simulink model "uwb_re_blackbox"  (Simulink 8.0)
settings: Solver=ode45  StartTime=0.0  StopTime=330  RelTol=1e-3
InitFcn:
  | set_channel;
  | Int_Data_input;
StopFcn:
  | abc=1;
undefined symbols (not defined in the file or in its folder): rsgenpoly
libraries: commutil2 x88, simulink x53, dspmtrx3 x33, dspindex x16, xbsIndex_r4 x12, commcnvcod2 x8, commblkcod2 x8, dspsigops x2, commsink2 x2, commchan3 x1
(part 3 of 5)

== system uwb_re_blackbox/Subsystem2/Transmit2/Spreading/Hop3 ==
  data : Inport
  s : Inport  Port=2
  Gain2 : Gain  Gain=-1  OutDataTypeStr=int8
  Gain4 : Gain  Gain=-1  OutDataTypeStr=int8
  Kron : Subsystem
      mask Display:
      | disp('KRON');
      | 
      | port_label('input',1,'P');
      | port_label('input',2,'-P');
      | port_label('input',3,'sel');
      | port_label('output',1,'burst');
  Kron1 : Subsystem
      mask Display:
      | disp('KRON');
      | 
      | port_label('input',1,'S');
      | port_label('input',2,'-S');
      | port_label('input',3,'sel');
      | port_label('output',1,'signS');
  Subsystem2 : Subsystem
      mask Display: disp('1/2 Frame data pulse')
  Subsystem3 : Subsystem
      mask Display:
      | port_label('input',1,'data_conv');
      | port_label('output',2,'sign');
      | port_label('output',1,'position');
  Subsystem5 : Subsystem
      mask Display:
      | disp('sel position');
      | 
      | port_label('input',1,'position');
      | port_label('input',2,'matrix');
      | port_label('output',1,'mat_po');
  p : Constant  Value=[-0.0022 -0.0103 -0.0386 -0.1133 -0.2542 -0.4160 -0.4388 -0.1363 0.4543 0.9559 0.9559 0.4543 -0.1363 -0.4388 -0.4160 -0.2542 -0.1133 -0.0386 -0.0103 -0.0022]*2^6  VectorParams1D=off  OutDataTypeStr=int8
      mask Display: disp('xung P')
  Hop1 : Outport
  wires:
  data/1 -> Subsystem3/1(In1)
  Subsystem5/1(Out1) -> Hop1/1
  Subsystem3/1(position) -> Subsystem5/1(In1)
  Subsystem2/1(Out1) -> Subsystem5/2(matrix)
  Subsystem3/2(sign) -> Kron1/3(sel)
  s/1 -> Gain2/1, Kron1/1(p)
  Kron/1(burst) -> Subsystem2/1(In1)
  p/1 -> Gain4/1, Kron/1(p)
  Kron1/1(burst) -> Kron/3(sel)
  Gain4/1 -> Kron/2(-p)
  Gain2/1 -> Kron1/2(-p)

== system uwb_re_blackbox/Subsystem2/Transmit2/Spreading/Hop4 ==
  data : Inport
  s : Inport  Port=2
  Gain2 : Gain  Gain=-1  OutDataTypeStr=int8
  Gain4 : Gain  Gain=-1  OutDataTypeStr=int8
  Kron : Subsystem
      mask Display:
      | disp('KRON');
      | 
      | port_label('input',1,'P');
      | port_label('input',2,'-P');
      | port_label('input',3,'sel');
      | port_label('output',1,'burst');
  Kron1 : Subsystem
      mask Display:
      | disp('KRON');
      | 
      | port_label('input',1,'S');
      | port_label('input',2,'-S');
      | port_label('input',3,'sel');
      | port_label('output',1,'signS');
  Subsystem2 : Subsystem
      mask Display: disp('1/2 Frame data pulse')
  Subsystem3 : Subsystem
      mask Display:
      | port_label('input',1,'data_conv');
      | port_label('output',2,'sign');
      | port_label('output',1,'position');
  Subsystem5 : Subsystem
      mask Display:
      | disp('sel position');
      | 
      | port_label('input',1,'position');
      | port_label('input',2,'matrix');
      | port_label('output',1,'mat_po');
  p : Constant  Value=[-0.0022 -0.0103 -0.0386 -0.1133 -0.2542 -0.4160 -0.4388 -0.1363 0.4543 0.9559 0.9559 0.4543 -0.1363 -0.4388 -0.4160 -0.2542 -0.1133 -0.0386 -0.0103 -0.0022]*2^6  VectorParams1D=off  OutDataTypeStr=int8
      mask Display: disp('xung P')
  Hop1 : Outport
  wires:
  Gain2/1 -> Kron1/2(-p)
  Gain4/1 -> Kron/2(-p)
  Kron1/1(burst) -> Kron/3(sel)
  p/1 -> Kron/1(p), Gain4/1
  Kron/1(burst) -> Subsystem2/1(In1)
  s/1 -> Kron1/1(p), Gain2/1
  Subsystem3/2(sign) -> Kron1/3(sel)
  Subsystem2/1(Out1) -> Subsystem5/2(matrix)
  Subsystem3/1(position) -> Subsystem5/1(In1)
  Subsystem5/1(Out1) -> Hop1/1
  data/1 -> Subsystem3/1(In1)

== system uwb_re_blackbox/Subsystem2/Transmit2/Spreading/Hop5 ==
  data : Inport
  s : Inport  Port=2
  Gain2 : Gain  Gain=-1  OutDataTypeStr=int8
  Gain4 : Gain  Gain=-1  OutDataTypeStr=int8
  Kron : Subsystem
      mask Display:
      | disp('KRON');
      | 
      | port_label('input',1,'P');
      | port_label('input',2,'-P');
      | port_label('input',3,'sel');
      | port_label('output',1,'burst');
  Kron1 : Subsystem
      mask Display:
      | disp('KRON');
      | 
      | port_label('input',1,'S');
      | port_label('input',2,'-S');
      | port_label('input',3,'sel');
      | port_label('output',1,'signS');
  Subsystem2 : Subsystem
      mask Display: disp('1/2 Frame data pulse')
  Subsystem3 : Subsystem
      mask Display:
      | port_label('input',1,'data_conv');
      | port_label('output',2,'sign');
      | port_label('output',1,'position');
  Subsystem5 : Subsystem
      mask Display:
      | disp('sel position');
      | 
      | port_label('input',1,'position');
      | port_label('input',2,'matrix');
      | port_label('output',1,'mat_po');
  p : Constant  Value=[-0.0022 -0.0103 -0.0386 -0.1133 -0.2542 -0.4160 -0.4388 -0.1363 0.4543 0.9559 0.9559 0.4543 -0.1363 -0.4388 -0.4160 -0.2542 -0.1133 -0.0386 -0.0103 -0.0022]*2^6  VectorParams1D=off  OutDataTypeStr=int8
      mask Display: disp('xung P')
  Hop1 : Outport
  wires:
  data/1 -> Subsystem3/1(In1)
  Subsystem5/1(Out1) -> Hop1/1
  Subsystem3/1(position) -> Subsystem5/1(In1)
  Subsystem2/1(Out1) -> Subsystem5/2(matrix)
  Subsystem3/2(sign) -> Kron1/3(sel)
  s/1 -> Gain2/1, Kron1/1(p)
  Kron/1(burst) -> Subsystem2/1(In1)
  p/1 -> Gain4/1, Kron/1(p)
  Kron1/1(burst) -> Kron/3(sel)
  Gain4/1 -> Kron/2(-p)
  Gain2/1 -> Kron1/2(-p)

== system uwb_re_blackbox/Subsystem2/Transmit2/Spreading/Hop6 ==
  data : Inport
  s : Inport  Port=2
  Gain2 : Gain  Gain=-1  OutDataTypeStr=int8
  Gain4 : Gain  Gain=-1  OutDataTypeStr=int8
  Kron : Subsystem
      mask Display:
      | disp('KRON');
      | 
      | port_label('input',1,'P');
      | port_label('input',2,'-P');
      | port_label('input',3,'sel');
      | port_label('output',1,'burst');
  Kron1 : Subsystem
      mask Display:
      | disp('KRON');
      | 
      | port_label('input',1,'S');
      | port_label('input',2,'-S');
      | port_label('input',3,'sel');
      | port_label('output',1,'signS');
  Subsystem2 : Subsystem
      mask Display: disp('1/2 Frame data pulse')
  Subsystem3 : Subsystem
      mask Display:
      | port_label('input',1,'data_conv');
      | port_label('output',2,'sign');
      | port_label('output',1,'position');
  Subsystem5 : Subsystem
      mask Display:
      | disp('sel position');
      | 
      | port_label('input',1,'position');
      | port_label('input',2,'matrix');
      | port_label('output',1,'mat_po');
  p : Constant  Value=[-0.0022 -0.0103 -0.0386 -0.1133 -0.2542 -0.4160 -0.4388 -0.1363 0.4543 0.9559 0.9559 0.4543 -0.1363 -0.4388 -0.4160 -0.2542 -0.1133 -0.0386 -0.0103 -0.0022]*2^6  VectorParams1D=off  OutDataTypeStr=int8
      mask Display: disp('xung P')
  Hop1 : Outport
  wires:
  Gain2/1 -> Kron1/2(-p)
  Gain4/1 -> Kron/2(-p)
  Kron1/1(burst) -> Kron/3(sel)
  p/1 -> Kron/1(p), Gain4/1
  Kron/1(burst) -> Subsystem2/1(In1)
  s/1 -> Kron1/1(p), Gain2/1
  Subsystem3/2(sign) -> Kron1/3(sel)
  Subsystem2/1(Out1) -> Subsystem5/2(matrix)
  Subsystem3/1(position) -> Subsystem5/1(In1)
  Subsystem5/1(Out1) -> Hop1/1
  data/1 -> Subsystem3/1(In1)

== system uwb_re_blackbox/Subsystem2/Transmit2/Spreading/Hop7 ==
  data : Inport
  s : Inport  Port=2
  Gain2 : Gain  Gain=-1  OutDataTypeStr=int8
  Gain4 : Gain  Gain=-1  OutDataTypeStr=int8
  Kron : Subsystem
      mask Display:
      | disp('KRON');
      | 
      | port_label('input',1,'P');
      | port_label('input',2,'-P');
      | port_label('input',3,'sel');
      | port_label('output',1,'burst');
  Kron1 : Subsystem
      mask Display:
      | disp('KRON');
      | 
      | port_label('input',1,'S');
      | port_label('input',2,'-S');
      | port_label('input',3,'sel');
      | port_label('output',1,'signS');
  Subsystem2 : Subsystem
      mask Display: disp('1/2 Frame data pulse')
  Subsystem3 : Subsystem
      mask Display:
      | port_label('input',1,'data_conv');
      | port_label('output',2,'sign');
      | port_label('output',1,'position');
  Subsystem5 : Subsystem
      mask Display:
      | disp('sel position');
      | 
      | port_label('input',1,'position');
      | port_label('input',2,'matrix');
      | port_label('output',1,'mat_po');
  p : Constant  Value=[-0.0022 -0.0103 -0.0386 -0.1133 -0.2542 -0.4160 -0.4388 -0.1363 0.4543 0.9559 0.9559 0.4543 -0.1363 -0.4388 -0.4160 -0.2542 -0.1133 -0.0386 -0.0103 -0.0022]*2^6  VectorParams1D=off  OutDataTypeStr=int8
      mask Display: disp('xung P')
  Hop1 : Outport
  wires:
  data/1 -> Subsystem3/1(In1)
  Subsystem5/1(Out1) -> Hop1/1
  Subsystem3/1(position) -> Subsystem5/1(In1)
  Subsystem2/1(Out1) -> Subsystem5/2(matrix)
  Subsystem3/2(sign) -> Kron1/3(sel)
  s/1 -> Gain2/1, Kron1/1(p)
  Kron/1(burst) -> Subsystem2/1(In1)
  p/1 -> Gain4/1, Kron/1(p)
  Kron1/1(burst) -> Kron/3(sel)
  Gain4/1 -> Kron/2(-p)
  Gain2/1 -> Kron1/2(-p)

== system uwb_re_blackbox/Subsystem2/Transmit2/Spreading/Hop8 ==
  data : Inport
  s : Inport  Port=2
  Gain2 : Gain  Gain=-1  OutDataTypeStr=int8
  Gain4 : Gain  Gain=-1  OutDataTypeStr=int8
  Kron : Subsystem
      mask Display:
      | disp('KRON');
      | 
      | port_label('input',1,'P');
      | port_label('input',2,'-P');
      | port_label('input',3,'sel');
      | port_label('output',1,'burst');
  Kron1 : Subsystem
      mask Display:
      | disp('KRON');
      | 
      | port_label('input',1,'S');
      | port_label('input',2,'-S');
      | port_label('input',3,'sel');
      | port_label('output',1,'signS');
  Subsystem2 : Subsystem
      mask Display: disp('1/2 Frame data pulse')
  Subsystem3 : Subsystem
      mask Display:
      | port_label('input',1,'data_conv');
      | port_label('output',2,'sign');
      | port_label('output',1,'position');
  Subsystem5 : Subsystem
      mask Display:
      | disp('sel position');
      | 
      | port_label('input',1,'position');
      | port_label('input',2,'matrix');
      | port_label('output',1,'mat_po');
  p : Constant  Value=[-0.0022 -0.0103 -0.0386 -0.1133 -0.2542 -0.4160 -0.4388 -0.1363 0.4543 0.9559 0.9559 0.4543 -0.1363 -0.4388 -0.4160 -0.2542 -0.1133 -0.0386 -0.0103 -0.0022]*2^6  VectorParams1D=off  OutDataTypeStr=int8
      mask Display: disp('xung P')
  Hop1 : Outport
  wires:
  Gain2/1 -> Kron1/2(-p)
  Gain4/1 -> Kron/2(-p)
  Kron1/1(burst) -> Kron/3(sel)
  p/1 -> Kron/1(p), Gain4/1
  Kron/1(burst) -> Subsystem2/1(In1)
  s/1 -> Kron1/1(p), Gain2/1
  Subsystem3/2(sign) -> Kron1/3(sel)
  Subsystem2/1(Out1) -> Subsystem5/2(matrix)
  Subsystem3/1(position) -> Subsystem5/1(In1)
  Subsystem5/1(Out1) -> Hop1/1
  data/1 -> Subsystem3/1(In1)

== system uwb_re_blackbox/Subsystem2/Transmit2/Spreading/Hop9 ==
  data : Inport
  s : Inport  Port=2
  Gain2 : Gain  Gain=-1  OutDataTypeStr=int8
  Gain4 : Gain  Gain=-1  OutDataTypeStr=int8
  Kron : Subsystem
      mask Display:
      | disp('KRON');
      | 
      | port_label('input',1,'P');
      | port_label('input',2,'-P');
      | port_label('input',3,'sel');
      | port_label('output',1,'burst');
  Kron1 : Subsystem
      mask Display:
      | disp('KRON');
      | 
      | port_label('input',1,'S');
      | port_label('input',2,'-S');
      | port_label('input',3,'sel');
      | port_label('output',1,'signS');
  Subsystem2 : Subsystem
      mask Display: disp('1/2 Frame data pulse')
  Subsystem3 : Subsystem
      mask Display:
      | port_label('input',1,'data_conv');
      | port_label('output',2,'sign');
      | port_label('output',1,'position');
  Subsystem5 : Subsystem
      mask Display:
      | disp('sel position');
      | 
      | port_label('input',1,'position');
      | port_label('input',2,'matrix');
      | port_label('output',1,'mat_po');
  p : Constant  Value=[-0.0022 -0.0103 -0.0386 -0.1133 -0.2542 -0.4160 -0.4388 -0.1363 0.4543 0.9559 0.9559 0.4543 -0.1363 -0.4388 -0.4160 -0.2542 -0.1133 -0.0386 -0.0103 -0.0022]*2^6  VectorParams1D=off  OutDataTypeStr=int8
      mask Display: disp('xung P')
  Hop1 : Outport
  wires:
  data/1 -> Subsystem3/1(In1)
  Subsystem5/1(Out1) -> Hop1/1
  Subsystem3/1(position) -> Subsystem5/1(In1)
  Subsystem2/1(Out1) -> Subsystem5/2(matrix)
  Subsystem3/2(sign) -> Kron1/3(sel)
  s/1 -> Gain2/1, Kron1/1(p)
  Kron/1(burst) -> Subsystem2/1(In1)
  p/1 -> Gain4/1, Kron/1(p)
  Kron1/1(burst) -> Kron/3(sel)
  Gain4/1 -> Kron/2(-p)
  Gain2/1 -> Kron1/2(-p)

== system uwb_re_blackbox/Subsystem2/Creat n_re/delay transmition/Truyen Tre/Switch Case Action Subsystem ==
  In1 : Inport
  Action Port : ActionPort  ActionType=case
  Out1 : Outport
  wires:
  In1/1 -> Out1/1

== system uwb_re_blackbox/Subsystem2/Creat n_re/delay transmition/Truyen Tre/Switch Case Action Subsystem1 ==
  In1 : Inport
  Action Port : ActionPort  ActionType=default
  Out1 : Outport
  wires:
  In1/1 -> Out1/1

== system uwb_re_blackbox/Subsystem2/Creat n_re/delay transmition/Truyen Tre chuc/Switch Case Action Subsystem ==
  In1 : Inport
  Action Port : ActionPort  ActionType=case
  Out1 : Outport
  wires:
  In1/1 -> Out1/1

== system uwb_re_blackbox/Subsystem2/Creat n_re/delay transmition/Truyen Tre chuc/Switch Case Action Subsystem1 ==
  In1 : Inport
  Action Port : ActionPort  ActionType=case
  Out1 : Outport
  wires:
  In1/1 -> Out1/1

== system uwb_re_blackbox/Subsystem2/Creat n_re/delay transmition/Truyen Tre chuc/Switch Case Action Subsystem2 ==
  In1 : Inport
  Action Port : ActionPort  ActionType=case
  Out1 : Outport
  wires:
  In1/1 -> Out1/1

== system uwb_re_blackbox/Subsystem2/Creat n_re/delay transmition/Truyen Tre chuc/Switch Case Action Subsystem3 ==
  In1 : Inport
  Action Port : ActionPort  ActionType=case
  Out1 : Outport
  wires:
  In1/1 -> Out1/1

== system uwb_re_blackbox/Subsystem2/Creat n_re/delay transmition/Truyen Tre chuc/Switch Case Action Subsystem4 ==
  In1 : Inport
  Action Port : ActionPort  ActionType=case
  Out1 : Outport
  wires:
  In1/1 -> Out1/1

== system uwb_re_blackbox/Subsystem2/Creat n_re/delay transmition/Truyen Tre chuc/Switch Case Action Subsystem5 ==
  In1 : Inport
  Action Port : ActionPort  ActionType=case
  Out1 : Outport
  wires:
  In1/1 -> Out1/1

== system uwb_re_blackbox/Subsystem2/Creat n_re/delay transmition/Truyen Tre chuc/Switch Case Action Subsystem6 ==
  In1 : Inport
  Action Port : ActionPort  ActionType=case
  Out1 : Outport
  wires:
  In1/1 -> Out1/1

== system uwb_re_blackbox/Subsystem2/Creat n_re/delay transmition/Truyen Tre chuc/Switch Case Action Subsystem7 ==
  In1 : Inport
  Action Port : ActionPort  ActionType=case
  Out1 : Outport
  wires:
  In1/1 -> Out1/1

== system uwb_re_blackbox/Subsystem2/Creat n_re/delay transmition/Truyen Tre chuc/Switch Case Action Subsystem8 ==
  In1 : Inport
  Action Port : ActionPort  ActionType=case
  Out1 : Outport
  wires:
  In1/1 -> Out1/1

== system uwb_re_blackbox/Subsystem2/Creat n_re/delay transmition/Truyen Tre chuc/Switch Case Action Subsystem9 ==
  In1 : Inport
  Action Port : ActionPort  ActionType=default
  Out1 : Outport
  wires:
  In1/1 -> Out1/1

== system uwb_re_blackbox/Subsystem2/Creat n_re/delay transmition/Truyen Tre don vi/Switch Case Action Subsystem ==
  In1 : Inport
  Action Port : ActionPort  ActionType=case
  Out1 : Outport
  wires:
  In1/1 -> Out1/1

== system uwb_re_blackbox/Subsystem2/Creat n_re/delay transmition/Truyen Tre don vi/Switch Case Action Subsystem1 ==
  In1 : Inport
  Action Port : ActionPort  ActionType=case
  Out1 : Outport
  wires:
  In1/1 -> Out1/1

== system uwb_re_blackbox/Subsystem2/Creat n_re/delay transmition/Truyen Tre don vi/Switch Case Action Subsystem2 ==
  In1 : Inport
  Action Port : ActionPort  ActionType=case
  Out1 : Outport
  wires:
  In1/1 -> Out1/1

== system uwb_re_blackbox/Subsystem2/Creat n_re/delay transmition/Truyen Tre don vi/Switch Case Action Subsystem3 ==
  In1 : Inport
  Action Port : ActionPort  ActionType=case
  Out1 : Outport
  wires:
  In1/1 -> Out1/1

== system uwb_re_blackbox/Subsystem2/Creat n_re/delay transmition/Truyen Tre don vi/Switch Case Action Subsystem4 ==
  In1 : Inport
  Action Port : ActionPort  ActionType=case
  Out1 : Outport
  wires:
  In1/1 -> Out1/1

== system uwb_re_blackbox/Subsystem2/Creat n_re/delay transmition/Truyen Tre don vi/Switch Case Action Subsystem5 ==
  In1 : Inport
  Action Port : ActionPort  ActionType=case
  Out1 : Outport
  wires:
  In1/1 -> Out1/1

== system uwb_re_blackbox/Subsystem2/Creat n_re/delay transmition/Truyen Tre don vi/Switch Case Action Subsystem6 ==
  In1 : Inport
  Action Port : ActionPort  ActionType=case
  Out1 : Outport
  wires:
  In1/1 -> Out1/1

== system uwb_re_blackbox/Subsystem2/Creat n_re/delay transmition/Truyen Tre don vi/Switch Case Action Subsystem7 ==
  In1 : Inport
  Action Port : ActionPort  ActionType=case
  Out1 : Outport
  wires:
  In1/1 -> Out1/1

== system uwb_re_blackbox/Subsystem2/Creat n_re/delay transmition/Truyen Tre don vi/Switch Case Action Subsystem8 ==
  In1 : Inport
  Action Port : ActionPort  ActionType=case
  Out1 : Outport
  wires:
  In1/1 -> Out1/1

== system uwb_re_blackbox/Subsystem2/Creat n_re/delay transmition/Truyen Tre don vi/Switch Case Action Subsystem9 ==
  In1 : Inport
  Action Port : ActionPort  ActionType=default
  Out1 : Outport
  wires:
  In1/1 -> Out1/1

== system uwb_re_blackbox/Subsystem2/Creat n_re/delay transmition/Truyen Tre tram/Switch Case Action Subsystem ==
  In1 : Inport
  Action Port : ActionPort  ActionType=case
  Out1 : Outport
  wires:
  In1/1 -> Out1/1

== system uwb_re_blackbox/Subsystem2/Creat n_re/delay transmition/Truyen Tre tram/Switch Case Action Subsystem1 ==
  In1 : Inport
  Action Port : ActionPort  ActionType=case
  Out1 : Outport
  wires:
  In1/1 -> Out1/1

== system uwb_re_blackbox/Subsystem2/Creat n_re/delay transmition/Truyen Tre tram/Switch Case Action Subsystem2 ==
  In1 : Inport
  Action Port : ActionPort  ActionType=case
  Out1 : Outport
  wires:
  In1/1 -> Out1/1

== system uwb_re_blackbox/Subsystem2/Creat n_re/delay transmition/Truyen Tre tram/Switch Case Action Subsystem3 ==
  In1 : Inport
  Action Port : ActionPort  ActionType=case
  Out1 : Outport
  wires:
  In1/1 -> Out1/1

== system uwb_re_blackbox/Subsystem2/Creat n_re/delay transmition/Truyen Tre tram/Switch Case Action Subsystem4 ==
  In1 : Inport
  Action Port : ActionPort  ActionType=case
  Out1 : Outport
  wires:
  In1/1 -> Out1/1

== system uwb_re_blackbox/Subsystem2/Creat n_re/delay transmition/Truyen Tre tram/Switch Case Action Subsystem5 ==
  In1 : Inport
  Action Port : ActionPort  ActionType=case
  Out1 : Outport
  wires:
  In1/1 -> Out1/1

== system uwb_re_blackbox/Subsystem2/Creat n_re/delay transmition/Truyen Tre tram/Switch Case Action Subsystem6 ==
  In1 : Inport
  Action Port : ActionPort  ActionType=case
  Out1 : Outport
  wires:
  In1/1 -> Out1/1

== system uwb_re_blackbox/Subsystem2/Creat n_re/delay transmition/Truyen Tre tram/Switch Case Action Subsystem7 ==
  In1 : Inport
  Action Port : ActionPort  ActionType=case
  Out1 : Outport
  wires:
  In1/1 -> Out1/1

== system uwb_re_blackbox/Subsystem2/Creat n_re/delay transmition/Truyen Tre tram/Switch Case Action Subsystem8 ==
  In1 : Inport
  Action Port : ActionPort  ActionType=case
  Out1 : Outport
  wires:
  In1/1 -> Out1/1

== system uwb_re_blackbox/Subsystem2/Creat n_re/delay transmition/Truyen Tre tram/Switch Case Action Subsystem9 ==
  In1 : Inport
  Action Port : ActionPort  ActionType=default
  Out1 : Outport
  wires:
  In1/1 -> Out1/1

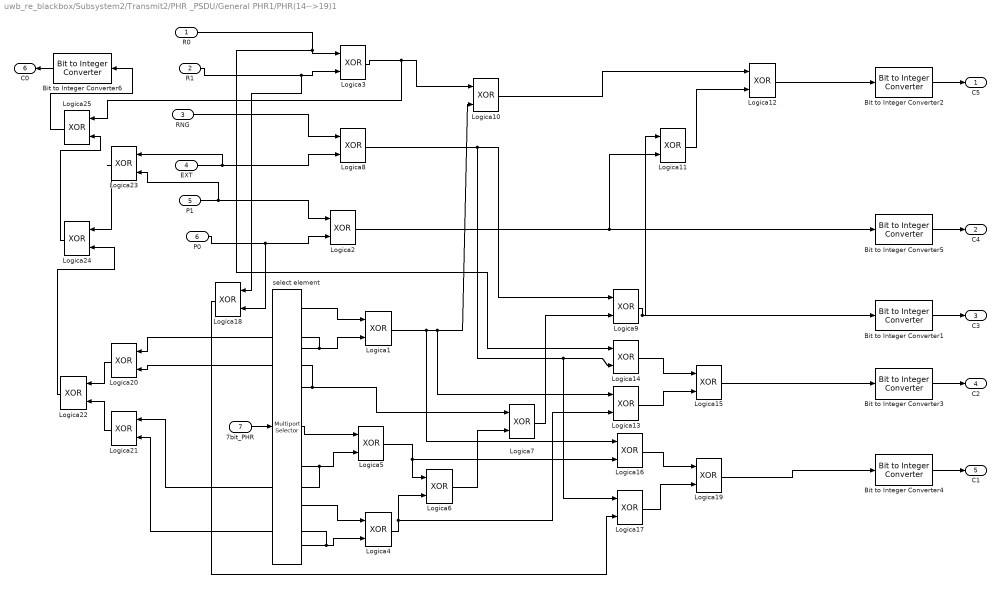
== system uwb_re_blackbox/Subsystem2/Transmit2/PHR _PSDU/General PHR1/PHR(14-->19)1 ==
  R0 : Inport
  R1 : Inport  Port=2
  RNG : Inport  Port=3
  EXT : Inport  Port=4
  P1 : Inport  Port=5
  P0 : Inport  Port=6
  7bit_PHR : Inport  Port=7
  Bit to Integer Converter{1..6} (6 alike) : commutil2/Bit to Integer Converter  nbits=1  bitOrder=MSB first  signedOutputValues=Unsigned  outDtype=int8  outDtypeSigned=Inherit via internal rule
  Logica{1..25} (25 alike) : Logic  Operator=XOR  AllPortsSameDT=off  OutDataTypeStr=boolean
  select element : dspindex/Multiport Selector  rowsOrCols=Columns  idxCellArray={ 1,2,3,4,5,6,7}  idxErrMode=Clip Index
  C5 : Outport
  C4 : Outport  Port=2
  C3 : Outport  Port=3
  C2 : Outport  Port=4
  C1 : Outport  Port=5
  C0 : Outport  Port=6
  wires:
  Logica25/1 -> Bit to Integer Converter6/1
  Logica24/1 -> Logica25/2
  Logica22/1 -> Logica24/2
  Logica23/1 -> Logica24/1
  Logica21/1 -> Logica22/2
  Logica20/1 -> Logica22/1
  Bit to Integer Converter6/1 -> C0/1
  Logica19/1 -> Bit to Integer Converter4/1
  Logica17/1 -> Logica19/2
  Logica16/1 -> Logica19/1
  Logica18/1 -> Logica17/2
  Bit to Integer Converter4/1 -> C1/1
  Logica15/1 -> Bit to Integer Converter3/1
  Logica13/1 -> Logica15/2
  Logica14/1 -> Logica15/1
  Bit to Integer Converter3/1 -> C2/1
  Logica12/1 -> Bit to Integer Converter2/1
  Logica11/1 -> Logica12/2
  Logica10/1 -> Logica12/1
  Logica1/1 -> Logica16/1, Logica13/1, Logica10/2
  Logica3/1 -> Logica25/1, Logica10/1
  Logica9/1 -> Logica11/1, Bit to Integer Converter1/1
  Logica7/1 -> Logica9/2
  Logica8/1 -> Logica17/1, Logica14/2, Logica9/1
  Bit to Integer Converter1/1 -> C3/1
  EXT/1 -> Logica23/1, Logica8/2
  RNG/1 -> Logica8/1
  Logica6/1 -> Logica7/2
  select element/3 -> Logica20/2, Logica7/1
  Logica4/1 -> Logica13/2, Logica6/2
  Logica5/1 -> Logica16/2, Logica6/1
  select element/5 -> Logica21/1, Logica5/2
  select element/4 -> Logica5/1
  select element/7 -> Logica21/2, Logica4/2
  select element/6 -> Logica4/1
  Logica2/1 -> Logica11/2, Bit to Integer Converter5/1
  P0/1 -> Logica18/2, Logica2/2
  P1/1 -> Logica23/2, Logica2/1
  select element/2 -> Logica20/1, Logica1/2
  select element/1 -> Logica1/1
  R1/1 -> Logica18/1, Logica3/2
  R0/1 -> Logica14/1, Logica3/1
  7bit_PHR/1 -> select element/1
  Bit to Integer Converter5/1 -> C4/1
  Bit to Integer Converter2/1 -> C5/1

== system uwb_re_blackbox/Subsystem2/Transmit2/PHR _PSDU/General PHR1/de2bi ==
  Noctet : Inport
  Integer to Bit Converter : commutil2/Integer to Bit Converter  nbits=7  signedInputValues=Unsigned  bitOrder=MSB first  outDtype=int8
  Transpose : dspmtrx3/Transpose  Hermitian=off  overflowFlag=off
  7bit_PHR : Outport
  wires:
  Transpose/1 -> 7bit_PHR/1
  Noctet/1 -> Integer to Bit Converter/1
  Integer to Bit Converter/1 -> Transpose/1

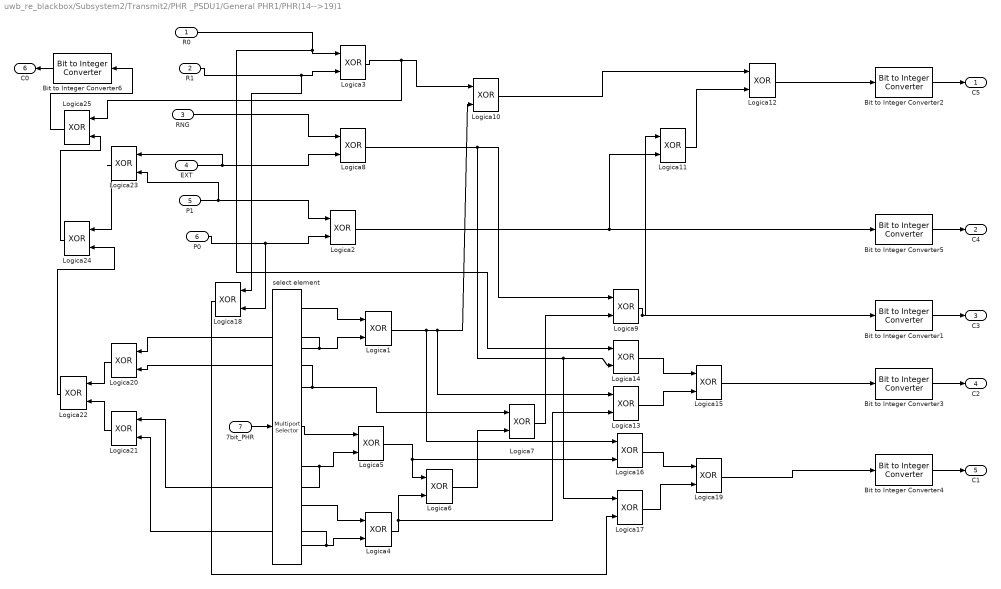
== system uwb_re_blackbox/Subsystem2/Transmit2/PHR _PSDU1/General PHR1/PHR(14-->19)1 ==
  R0 : Inport
  R1 : Inport  Port=2
  RNG : Inport  Port=3
  EXT : Inport  Port=4
  P1 : Inport  Port=5
  P0 : Inport  Port=6
  7bit_PHR : Inport  Port=7
  Bit to Integer Converter{1..6} (6 alike) : commutil2/Bit to Integer Converter  nbits=1  bitOrder=MSB first  signedOutputValues=Unsigned  outDtype=int8  outDtypeSigned=Inherit via internal rule
  Logica{1..25} (25 alike) : Logic  Operator=XOR  AllPortsSameDT=off  OutDataTypeStr=boolean
  select element : dspindex/Multiport Selector  rowsOrCols=Columns  idxCellArray={ 1,2,3,4,5,6,7}  idxErrMode=Clip Index
  C5 : Outport
  C4 : Outport  Port=2
  C3 : Outport  Port=3
  C2 : Outport  Port=4
  C1 : Outport  Port=5
  C0 : Outport  Port=6
  wires:
  Bit to Integer Converter2/1 -> C5/1
  Bit to Integer Converter5/1 -> C4/1
  7bit_PHR/1 -> select element/1
  R0/1 -> Logica3/1, Logica14/1
  R1/1 -> Logica3/2, Logica18/1
  select element/1 -> Logica1/1
  select element/2 -> Logica1/2, Logica20/1
  P1/1 -> Logica2/1, Logica23/2
  P0/1 -> Logica2/2, Logica18/2
  Logica2/1 -> Bit to Integer Converter5/1, Logica11/2
  select element/6 -> Logica4/1
  select element/7 -> Logica4/2, Logica21/2
  select element/4 -> Logica5/1
  select element/5 -> Logica5/2, Logica21/1
  Logica5/1 -> Logica6/1, Logica16/2
  Logica4/1 -> Logica6/2, Logica13/2
  select element/3 -> Logica7/1, Logica20/2
  Logica6/1 -> Logica7/2
  RNG/1 -> Logica8/1
  EXT/1 -> Logica8/2, Logica23/1
  Bit to Integer Converter1/1 -> C3/1
  Logica8/1 -> Logica9/1, Logica14/2, Logica17/1
  Logica7/1 -> Logica9/2
  Logica9/1 -> Bit to Integer Converter1/1, Logica11/1
  Logica3/1 -> Logica10/1, Logica25/1
  Logica1/1 -> Logica10/2, Logica13/1, Logica16/1
  Logica10/1 -> Logica12/1
  Logica11/1 -> Logica12/2
  Logica12/1 -> Bit to Integer Converter2/1
  Bit to Integer Converter3/1 -> C2/1
  Logica14/1 -> Logica15/1
  Logica13/1 -> Logica15/2
  Logica15/1 -> Bit to Integer Converter3/1
  Bit to Integer Converter4/1 -> C1/1
  Logica18/1 -> Logica17/2
  Logica16/1 -> Logica19/1
  Logica17/1 -> Logica19/2
  Logica19/1 -> Bit to Integer Converter4/1
  Bit to Integer Converter6/1 -> C0/1
  Logica20/1 -> Logica22/1
  Logica21/1 -> Logica22/2
  Logica23/1 -> Logica24/1
  Logica22/1 -> Logica24/2
  Logica24/1 -> Logica25/2
  Logica25/1 -> Bit to Integer Converter6/1

== system uwb_re_blackbox/Subsystem2/Transmit2/PHR _PSDU1/General PHR1/de2bi ==
  Noctet : Inport
  Integer to Bit Converter : commutil2/Integer to Bit Converter  nbits=7  signedInputValues=Unsigned  bitOrder=MSB first  outDtype=int8
  Transpose : dspmtrx3/Transpose  Hermitian=off  overflowFlag=off
  7bit_PHR : Outport
  wires:
  Integer to Bit Converter/1 -> Transpose/1
  Noctet/1 -> Integer to Bit Converter/1
  Transpose/1 -> 7bit_PHR/1

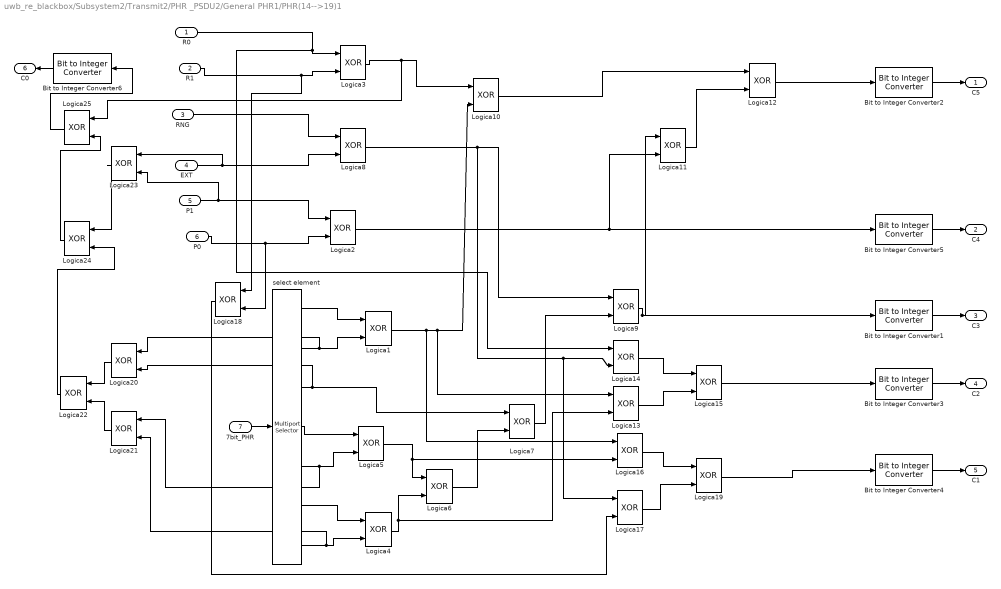
== system uwb_re_blackbox/Subsystem2/Transmit2/PHR _PSDU2/General PHR1/PHR(14-->19)1 ==
  R0 : Inport
  R1 : Inport  Port=2
  RNG : Inport  Port=3
  EXT : Inport  Port=4
  P1 : Inport  Port=5
  P0 : Inport  Port=6
  7bit_PHR : Inport  Port=7
  Bit to Integer Converter{1..6} (6 alike) : commutil2/Bit to Integer Converter  nbits=1  bitOrder=MSB first  signedOutputValues=Unsigned  outDtype=int8  outDtypeSigned=Inherit via internal rule
  Logica{1..25} (25 alike) : Logic  Operator=XOR  AllPortsSameDT=off  OutDataTypeStr=boolean
  select element : dspindex/Multiport Selector  rowsOrCols=Columns  idxCellArray={ 1,2,3,4,5,6,7}  idxErrMode=Clip Index
  C5 : Outport
  C4 : Outport  Port=2
  C3 : Outport  Port=3
  C2 : Outport  Port=4
  C1 : Outport  Port=5
  C0 : Outport  Port=6
  wires:
  Logica25/1 -> Bit to Integer Converter6/1
  Logica24/1 -> Logica25/2
  Logica22/1 -> Logica24/2
  Logica23/1 -> Logica24/1
  Logica21/1 -> Logica22/2
  Logica20/1 -> Logica22/1
  Bit to Integer Converter6/1 -> C0/1
  Logica19/1 -> Bit to Integer Converter4/1
  Logica17/1 -> Logica19/2
  Logica16/1 -> Logica19/1
  Logica18/1 -> Logica17/2
  Bit to Integer Converter4/1 -> C1/1
  Logica15/1 -> Bit to Integer Converter3/1
  Logica13/1 -> Logica15/2
  Logica14/1 -> Logica15/1
  Bit to Integer Converter3/1 -> C2/1
  Logica12/1 -> Bit to Integer Converter2/1
  Logica11/1 -> Logica12/2
  Logica10/1 -> Logica12/1
  Logica1/1 -> Logica16/1, Logica13/1, Logica10/2
  Logica3/1 -> Logica25/1, Logica10/1
  Logica9/1 -> Logica11/1, Bit to Integer Converter1/1
  Logica7/1 -> Logica9/2
  Logica8/1 -> Logica17/1, Logica14/2, Logica9/1
  Bit to Integer Converter1/1 -> C3/1
  EXT/1 -> Logica23/1, Logica8/2
  RNG/1 -> Logica8/1
  Logica6/1 -> Logica7/2
  select element/3 -> Logica20/2, Logica7/1
  Logica4/1 -> Logica13/2, Logica6/2
  Logica5/1 -> Logica16/2, Logica6/1
  select element/5 -> Logica21/1, Logica5/2
  select element/4 -> Logica5/1
  select element/7 -> Logica21/2, Logica4/2
  select element/6 -> Logica4/1
  Logica2/1 -> Logica11/2, Bit to Integer Converter5/1
  P0/1 -> Logica18/2, Logica2/2
  P1/1 -> Logica23/2, Logica2/1
  select element/2 -> Logica20/1, Logica1/2
  select element/1 -> Logica1/1
  R1/1 -> Logica18/1, Logica3/2
  R0/1 -> Logica14/1, Logica3/1
  7bit_PHR/1 -> select element/1
  Bit to Integer Converter5/1 -> C4/1
  Bit to Integer Converter2/1 -> C5/1

== system uwb_re_blackbox/Subsystem2/Transmit2/PHR _PSDU2/General PHR1/de2bi ==
  Noctet : Inport
  Integer to Bit Converter : commutil2/Integer to Bit Converter  nbits=7  signedInputValues=Unsigned  bitOrder=MSB first  outDtype=int8
  Transpose : dspmtrx3/Transpose  Hermitian=off  overflowFlag=off
  7bit_PHR : Outport
  wires:
  Transpose/1 -> 7bit_PHR/1
  Noctet/1 -> Integer to Bit Converter/1
  Integer to Bit Converter/1 -> Transpose/1

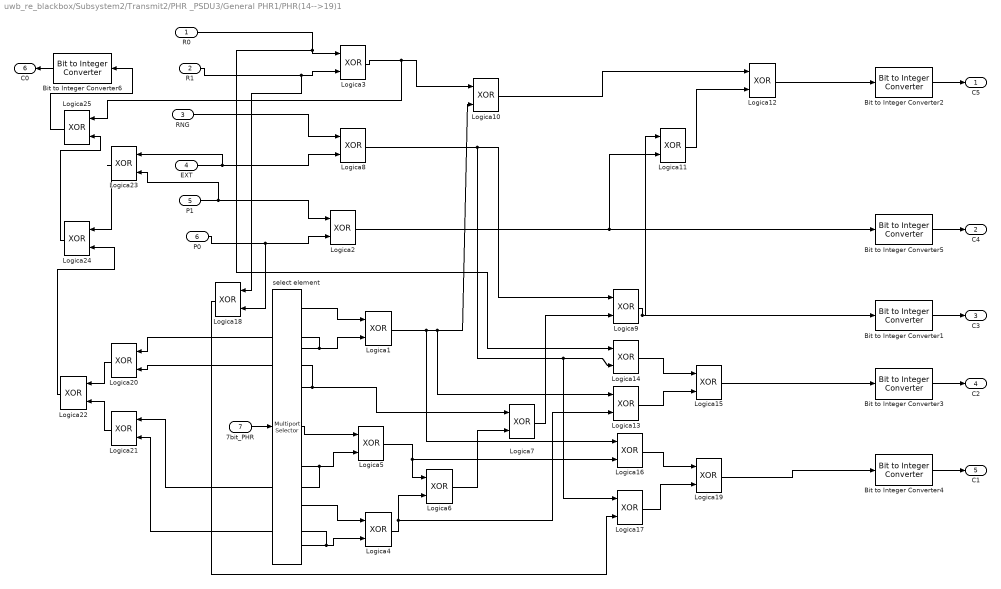
== system uwb_re_blackbox/Subsystem2/Transmit2/PHR _PSDU3/General PHR1/PHR(14-->19)1 ==
  R0 : Inport
  R1 : Inport  Port=2
  RNG : Inport  Port=3
  EXT : Inport  Port=4
  P1 : Inport  Port=5
  P0 : Inport  Port=6
  7bit_PHR : Inport  Port=7
  Bit to Integer Converter{1..6} (6 alike) : commutil2/Bit to Integer Converter  nbits=1  bitOrder=MSB first  signedOutputValues=Unsigned  outDtype=int8  outDtypeSigned=Inherit via internal rule
  Logica{1..25} (25 alike) : Logic  Operator=XOR  AllPortsSameDT=off  OutDataTypeStr=boolean
  select element : dspindex/Multiport Selector  rowsOrCols=Columns  idxCellArray={ 1,2,3,4,5,6,7}  idxErrMode=Clip Index
  C5 : Outport
  C4 : Outport  Port=2
  C3 : Outport  Port=3
  C2 : Outport  Port=4
  C1 : Outport  Port=5
  C0 : Outport  Port=6
  wires:
  Bit to Integer Converter2/1 -> C5/1
  Bit to Integer Converter5/1 -> C4/1
  7bit_PHR/1 -> select element/1
  R0/1 -> Logica3/1, Logica14/1
  R1/1 -> Logica3/2, Logica18/1
  select element/1 -> Logica1/1
  select element/2 -> Logica1/2, Logica20/1
  P1/1 -> Logica2/1, Logica23/2
  P0/1 -> Logica2/2, Logica18/2
  Logica2/1 -> Bit to Integer Converter5/1, Logica11/2
  select element/6 -> Logica4/1
  select element/7 -> Logica4/2, Logica21/2
  select element/4 -> Logica5/1
  select element/5 -> Logica5/2, Logica21/1
  Logica5/1 -> Logica6/1, Logica16/2
  Logica4/1 -> Logica6/2, Logica13/2
  select element/3 -> Logica7/1, Logica20/2
  Logica6/1 -> Logica7/2
  RNG/1 -> Logica8/1
  EXT/1 -> Logica8/2, Logica23/1
  Bit to Integer Converter1/1 -> C3/1
  Logica8/1 -> Logica9/1, Logica14/2, Logica17/1
  Logica7/1 -> Logica9/2
  Logica9/1 -> Bit to Integer Converter1/1, Logica11/1
  Logica3/1 -> Logica10/1, Logica25/1
  Logica1/1 -> Logica10/2, Logica13/1, Logica16/1
  Logica10/1 -> Logica12/1
  Logica11/1 -> Logica12/2
  Logica12/1 -> Bit to Integer Converter2/1
  Bit to Integer Converter3/1 -> C2/1
  Logica14/1 -> Logica15/1
  Logica13/1 -> Logica15/2
  Logica15/1 -> Bit to Integer Converter3/1
  Bit to Integer Converter4/1 -> C1/1
  Logica18/1 -> Logica17/2
  Logica16/1 -> Logica19/1
  Logica17/1 -> Logica19/2
  Logica19/1 -> Bit to Integer Converter4/1
  Bit to Integer Converter6/1 -> C0/1
  Logica20/1 -> Logica22/1
  Logica21/1 -> Logica22/2
  Logica23/1 -> Logica24/1
  Logica22/1 -> Logica24/2
  Logica24/1 -> Logica25/2
  Logica25/1 -> Bit to Integer Converter6/1

== system uwb_re_blackbox/Subsystem2/Transmit2/PHR _PSDU3/General PHR1/de2bi ==
  Noctet : Inport
  Integer to Bit Converter : commutil2/Integer to Bit Converter  nbits=7  signedInputValues=Unsigned  bitOrder=MSB first  outDtype=int8
  Transpose : dspmtrx3/Transpose  Hermitian=off  overflowFlag=off
  7bit_PHR : Outport
  wires:
  Integer to Bit Converter/1 -> Transpose/1
  Noctet/1 -> Integer to Bit Converter/1
  Transpose/1 -> 7bit_PHR/1

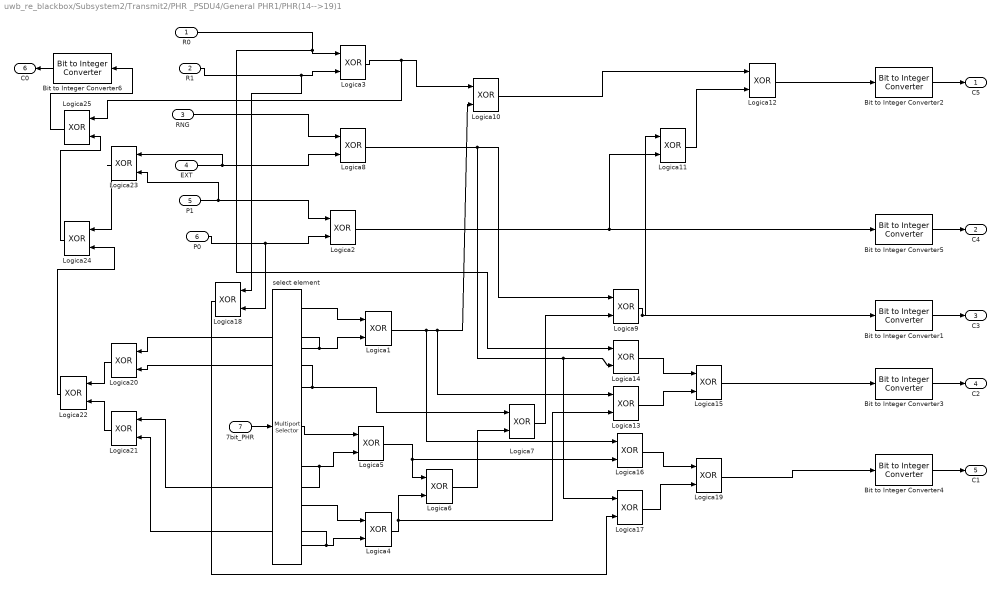
== system uwb_re_blackbox/Subsystem2/Transmit2/PHR _PSDU4/General PHR1/PHR(14-->19)1 ==
  R0 : Inport
  R1 : Inport  Port=2
  RNG : Inport  Port=3
  EXT : Inport  Port=4
  P1 : Inport  Port=5
  P0 : Inport  Port=6
  7bit_PHR : Inport  Port=7
  Bit to Integer Converter{1..6} (6 alike) : commutil2/Bit to Integer Converter  nbits=1  bitOrder=MSB first  signedOutputValues=Unsigned  outDtype=int8  outDtypeSigned=Inherit via internal rule
  Logica{1..25} (25 alike) : Logic  Operator=XOR  AllPortsSameDT=off  OutDataTypeStr=boolean
  select element : dspindex/Multiport Selector  rowsOrCols=Columns  idxCellArray={ 1,2,3,4,5,6,7}  idxErrMode=Clip Index
  C5 : Outport
  C4 : Outport  Port=2
  C3 : Outport  Port=3
  C2 : Outport  Port=4
  C1 : Outport  Port=5
  C0 : Outport  Port=6
  wires:
  Bit to Integer Converter2/1 -> C5/1
  Bit to Integer Converter5/1 -> C4/1
  7bit_PHR/1 -> select element/1
  R0/1 -> Logica3/1, Logica14/1
  R1/1 -> Logica3/2, Logica18/1
  select element/1 -> Logica1/1
  select element/2 -> Logica1/2, Logica20/1
  P1/1 -> Logica2/1, Logica23/2
  P0/1 -> Logica2/2, Logica18/2
  Logica2/1 -> Bit to Integer Converter5/1, Logica11/2
  select element/6 -> Logica4/1
  select element/7 -> Logica4/2, Logica21/2
  select element/4 -> Logica5/1
  select element/5 -> Logica5/2, Logica21/1
  Logica5/1 -> Logica6/1, Logica16/2
  Logica4/1 -> Logica6/2, Logica13/2
  select element/3 -> Logica7/1, Logica20/2
  Logica6/1 -> Logica7/2
  RNG/1 -> Logica8/1
  EXT/1 -> Logica8/2, Logica23/1
  Bit to Integer Converter1/1 -> C3/1
  Logica8/1 -> Logica9/1, Logica14/2, Logica17/1
  Logica7/1 -> Logica9/2
  Logica9/1 -> Bit to Integer Converter1/1, Logica11/1
  Logica3/1 -> Logica10/1, Logica25/1
  Logica1/1 -> Logica10/2, Logica13/1, Logica16/1
  Logica10/1 -> Logica12/1
  Logica11/1 -> Logica12/2
  Logica12/1 -> Bit to Integer Converter2/1
  Bit to Integer Converter3/1 -> C2/1
  Logica14/1 -> Logica15/1
  Logica13/1 -> Logica15/2
  Logica15/1 -> Bit to Integer Converter3/1
  Bit to Integer Converter4/1 -> C1/1
  Logica18/1 -> Logica17/2
  Logica16/1 -> Logica19/1
  Logica17/1 -> Logica19/2
  Logica19/1 -> Bit to Integer Converter4/1
  Bit to Integer Converter6/1 -> C0/1
  Logica20/1 -> Logica22/1
  Logica21/1 -> Logica22/2
  Logica23/1 -> Logica24/1
  Logica22/1 -> Logica24/2
  Logica24/1 -> Logica25/2
  Logica25/1 -> Bit to Integer Converter6/1

== system uwb_re_blackbox/Subsystem2/Transmit2/PHR _PSDU4/General PHR1/de2bi ==
  Noctet : Inport
  Integer to Bit Converter : commutil2/Integer to Bit Converter  nbits=7  signedInputValues=Unsigned  bitOrder=MSB first  outDtype=int8
  Transpose : dspmtrx3/Transpose  Hermitian=off  overflowFlag=off
  7bit_PHR : Outport
  wires:
  Integer to Bit Converter/1 -> Transpose/1
  Noctet/1 -> Integer to Bit Converter/1
  Transpose/1 -> 7bit_PHR/1

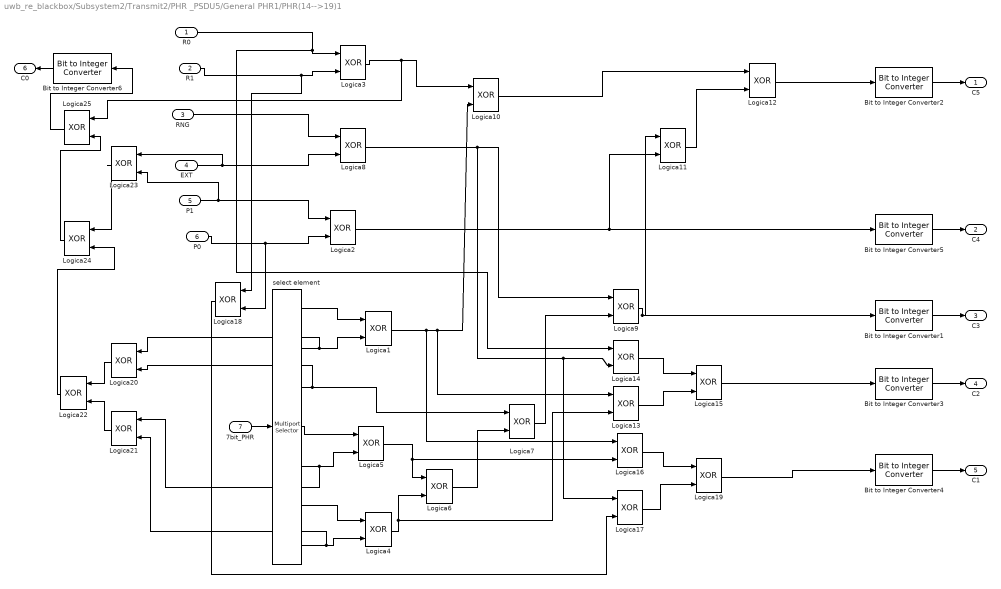
== system uwb_re_blackbox/Subsystem2/Transmit2/PHR _PSDU5/General PHR1/PHR(14-->19)1 ==
  R0 : Inport
  R1 : Inport  Port=2
  RNG : Inport  Port=3
  EXT : Inport  Port=4
  P1 : Inport  Port=5
  P0 : Inport  Port=6
  7bit_PHR : Inport  Port=7
  Bit to Integer Converter{1..6} (6 alike) : commutil2/Bit to Integer Converter  nbits=1  bitOrder=MSB first  signedOutputValues=Unsigned  outDtype=int8  outDtypeSigned=Inherit via internal rule
  Logica{1..25} (25 alike) : Logic  Operator=XOR  AllPortsSameDT=off  OutDataTypeStr=boolean
  select element : dspindex/Multiport Selector  rowsOrCols=Columns  idxCellArray={ 1,2,3,4,5,6,7}  idxErrMode=Clip Index
  C5 : Outport
  C4 : Outport  Port=2
  C3 : Outport  Port=3
  C2 : Outport  Port=4
  C1 : Outport  Port=5
  C0 : Outport  Port=6
  wires:
  Logica25/1 -> Bit to Integer Converter6/1
  Logica24/1 -> Logica25/2
  Logica22/1 -> Logica24/2
  Logica23/1 -> Logica24/1
  Logica21/1 -> Logica22/2
  Logica20/1 -> Logica22/1
  Bit to Integer Converter6/1 -> C0/1
  Logica19/1 -> Bit to Integer Converter4/1
  Logica17/1 -> Logica19/2
  Logica16/1 -> Logica19/1
  Logica18/1 -> Logica17/2
  Bit to Integer Converter4/1 -> C1/1
  Logica15/1 -> Bit to Integer Converter3/1
  Logica13/1 -> Logica15/2
  Logica14/1 -> Logica15/1
  Bit to Integer Converter3/1 -> C2/1
  Logica12/1 -> Bit to Integer Converter2/1
  Logica11/1 -> Logica12/2
  Logica10/1 -> Logica12/1
  Logica1/1 -> Logica16/1, Logica13/1, Logica10/2
  Logica3/1 -> Logica25/1, Logica10/1
  Logica9/1 -> Logica11/1, Bit to Integer Converter1/1
  Logica7/1 -> Logica9/2
  Logica8/1 -> Logica17/1, Logica14/2, Logica9/1
  Bit to Integer Converter1/1 -> C3/1
  EXT/1 -> Logica23/1, Logica8/2
  RNG/1 -> Logica8/1
  Logica6/1 -> Logica7/2
  select element/3 -> Logica20/2, Logica7/1
  Logica4/1 -> Logica13/2, Logica6/2
  Logica5/1 -> Logica16/2, Logica6/1
  select element/5 -> Logica21/1, Logica5/2
  select element/4 -> Logica5/1
  select element/7 -> Logica21/2, Logica4/2
  select element/6 -> Logica4/1
  Logica2/1 -> Logica11/2, Bit to Integer Converter5/1
  P0/1 -> Logica18/2, Logica2/2
  P1/1 -> Logica23/2, Logica2/1
  select element/2 -> Logica20/1, Logica1/2
  select element/1 -> Logica1/1
  R1/1 -> Logica18/1, Logica3/2
  R0/1 -> Logica14/1, Logica3/1
  7bit_PHR/1 -> select element/1
  Bit to Integer Converter5/1 -> C4/1
  Bit to Integer Converter2/1 -> C5/1

== system uwb_re_blackbox/Subsystem2/Transmit2/PHR _PSDU5/General PHR1/de2bi ==
  Noctet : Inport
  Integer to Bit Converter : commutil2/Integer to Bit Converter  nbits=7  signedInputValues=Unsigned  bitOrder=MSB first  outDtype=int8
  Transpose : dspmtrx3/Transpose  Hermitian=off  overflowFlag=off
  7bit_PHR : Outport
  wires:
  Transpose/1 -> 7bit_PHR/1
  Noctet/1 -> Integer to Bit Converter/1
  Integer to Bit Converter/1 -> Transpose/1

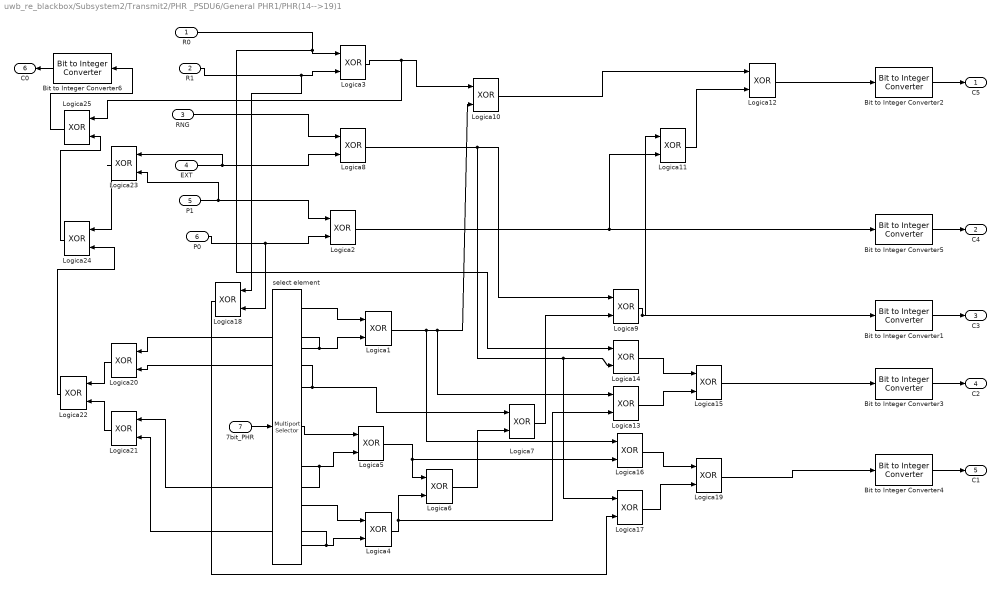
== system uwb_re_blackbox/Subsystem2/Transmit2/PHR _PSDU6/General PHR1/PHR(14-->19)1 ==
  R0 : Inport
  R1 : Inport  Port=2
  RNG : Inport  Port=3
  EXT : Inport  Port=4
  P1 : Inport  Port=5
  P0 : Inport  Port=6
  7bit_PHR : Inport  Port=7
  Bit to Integer Converter{1..6} (6 alike) : commutil2/Bit to Integer Converter  nbits=1  bitOrder=MSB first  signedOutputValues=Unsigned  outDtype=int8  outDtypeSigned=Inherit via internal rule
  Logica{1..25} (25 alike) : Logic  Operator=XOR  AllPortsSameDT=off  OutDataTypeStr=boolean
  select element : dspindex/Multiport Selector  rowsOrCols=Columns  idxCellArray={ 1,2,3,4,5,6,7}  idxErrMode=Clip Index
  C5 : Outport
  C4 : Outport  Port=2
  C3 : Outport  Port=3
  C2 : Outport  Port=4
  C1 : Outport  Port=5
  C0 : Outport  Port=6
  wires:
  Bit to Integer Converter2/1 -> C5/1
  Bit to Integer Converter5/1 -> C4/1
  7bit_PHR/1 -> select element/1
  R0/1 -> Logica3/1, Logica14/1
  R1/1 -> Logica3/2, Logica18/1
  select element/1 -> Logica1/1
  select element/2 -> Logica1/2, Logica20/1
  P1/1 -> Logica2/1, Logica23/2
  P0/1 -> Logica2/2, Logica18/2
  Logica2/1 -> Bit to Integer Converter5/1, Logica11/2
  select element/6 -> Logica4/1
  select element/7 -> Logica4/2, Logica21/2
  select element/4 -> Logica5/1
  select element/5 -> Logica5/2, Logica21/1
  Logica5/1 -> Logica6/1, Logica16/2
  Logica4/1 -> Logica6/2, Logica13/2
  select element/3 -> Logica7/1, Logica20/2
  Logica6/1 -> Logica7/2
  RNG/1 -> Logica8/1
  EXT/1 -> Logica8/2, Logica23/1
  Bit to Integer Converter1/1 -> C3/1
  Logica8/1 -> Logica9/1, Logica14/2, Logica17/1
  Logica7/1 -> Logica9/2
  Logica9/1 -> Bit to Integer Converter1/1, Logica11/1
  Logica3/1 -> Logica10/1, Logica25/1
  Logica1/1 -> Logica10/2, Logica13/1, Logica16/1
  Logica10/1 -> Logica12/1
  Logica11/1 -> Logica12/2
  Logica12/1 -> Bit to Integer Converter2/1
  Bit to Integer Converter3/1 -> C2/1
  Logica14/1 -> Logica15/1
  Logica13/1 -> Logica15/2
  Logica15/1 -> Bit to Integer Converter3/1
  Bit to Integer Converter4/1 -> C1/1
  Logica18/1 -> Logica17/2
  Logica16/1 -> Logica19/1
  Logica17/1 -> Logica19/2
  Logica19/1 -> Bit to Integer Converter4/1
  Bit to Integer Converter6/1 -> C0/1
  Logica20/1 -> Logica22/1
  Logica21/1 -> Logica22/2
  Logica23/1 -> Logica24/1
  Logica22/1 -> Logica24/2
  Logica24/1 -> Logica25/2
  Logica25/1 -> Bit to Integer Converter6/1

== system uwb_re_blackbox/Subsystem2/Transmit2/PHR _PSDU6/General PHR1/de2bi ==
  Noctet : Inport
  Integer to Bit Converter : commutil2/Integer to Bit Converter  nbits=7  signedInputValues=Unsigned  bitOrder=MSB first  outDtype=int8
  Transpose : dspmtrx3/Transpose  Hermitian=off  overflowFlag=off
  7bit_PHR : Outport
  wires:
  Integer to Bit Converter/1 -> Transpose/1
  Noctet/1 -> Integer to Bit Converter/1
  Transpose/1 -> 7bit_PHR/1

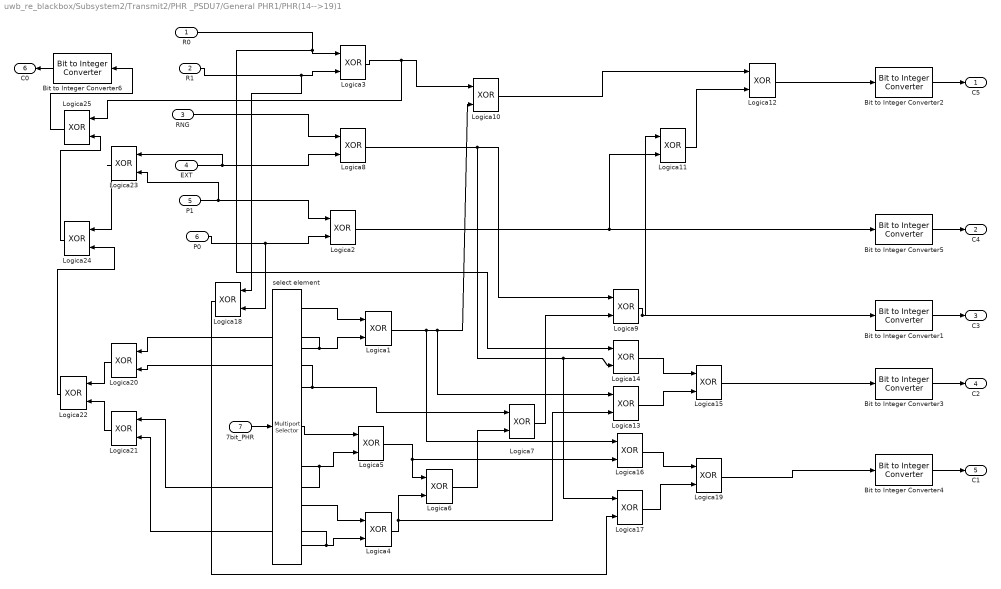
== system uwb_re_blackbox/Subsystem2/Transmit2/PHR _PSDU7/General PHR1/PHR(14-->19)1 ==
  R0 : Inport
  R1 : Inport  Port=2
  RNG : Inport  Port=3
  EXT : Inport  Port=4
  P1 : Inport  Port=5
  P0 : Inport  Port=6
  7bit_PHR : Inport  Port=7
  Bit to Integer Converter{1..6} (6 alike) : commutil2/Bit to Integer Converter  nbits=1  bitOrder=MSB first  signedOutputValues=Unsigned  outDtype=int8  outDtypeSigned=Inherit via internal rule
  Logica{1..25} (25 alike) : Logic  Operator=XOR  AllPortsSameDT=off  OutDataTypeStr=boolean
  select element : dspindex/Multiport Selector  rowsOrCols=Columns  idxCellArray={ 1,2,3,4,5,6,7}  idxErrMode=Clip Index
  C5 : Outport
  C4 : Outport  Port=2
  C3 : Outport  Port=3
  C2 : Outport  Port=4
  C1 : Outport  Port=5
  C0 : Outport  Port=6
  wires:
  Logica25/1 -> Bit to Integer Converter6/1
  Logica24/1 -> Logica25/2
  Logica22/1 -> Logica24/2
  Logica23/1 -> Logica24/1
  Logica21/1 -> Logica22/2
  Logica20/1 -> Logica22/1
  Bit to Integer Converter6/1 -> C0/1
  Logica19/1 -> Bit to Integer Converter4/1
  Logica17/1 -> Logica19/2
  Logica16/1 -> Logica19/1
  Logica18/1 -> Logica17/2
  Bit to Integer Converter4/1 -> C1/1
  Logica15/1 -> Bit to Integer Converter3/1
  Logica13/1 -> Logica15/2
  Logica14/1 -> Logica15/1
  Bit to Integer Converter3/1 -> C2/1
  Logica12/1 -> Bit to Integer Converter2/1
  Logica11/1 -> Logica12/2
  Logica10/1 -> Logica12/1
  Logica1/1 -> Logica16/1, Logica13/1, Logica10/2
  Logica3/1 -> Logica25/1, Logica10/1
  Logica9/1 -> Logica11/1, Bit to Integer Converter1/1
  Logica7/1 -> Logica9/2
  Logica8/1 -> Logica17/1, Logica14/2, Logica9/1
  Bit to Integer Converter1/1 -> C3/1
  EXT/1 -> Logica23/1, Logica8/2
  RNG/1 -> Logica8/1
  Logica6/1 -> Logica7/2
  select element/3 -> Logica20/2, Logica7/1
  Logica4/1 -> Logica13/2, Logica6/2
  Logica5/1 -> Logica16/2, Logica6/1
  select element/5 -> Logica21/1, Logica5/2
  select element/4 -> Logica5/1
  select element/7 -> Logica21/2, Logica4/2
  select element/6 -> Logica4/1
  Logica2/1 -> Logica11/2, Bit to Integer Converter5/1
  P0/1 -> Logica18/2, Logica2/2
  P1/1 -> Logica23/2, Logica2/1
  select element/2 -> Logica20/1, Logica1/2
  select element/1 -> Logica1/1
  R1/1 -> Logica18/1, Logica3/2
  R0/1 -> Logica14/1, Logica3/1
  7bit_PHR/1 -> select element/1
  Bit to Integer Converter5/1 -> C4/1
  Bit to Integer Converter2/1 -> C5/1

== system uwb_re_blackbox/Subsystem2/Transmit2/PHR _PSDU7/General PHR1/de2bi ==
  Noctet : Inport
  Integer to Bit Converter : commutil2/Integer to Bit Converter  nbits=7  signedInputValues=Unsigned  bitOrder=MSB first  outDtype=int8
  Transpose : dspmtrx3/Transpose  Hermitian=off  overflowFlag=off
  7bit_PHR : Outport
  wires:
  Transpose/1 -> 7bit_PHR/1
  Noctet/1 -> Integer to Bit Converter/1
  Integer to Bit Converter/1 -> Transpose/1

== system uwb_re_blackbox/Subsystem2/Transmit2/Spreading/Hop1/Kron ==
  p : Inport
  -p : Inport  Port=2
  sel : Inport  Port=3
  Compare To Zero : simulink/Logic and Bit Operations/Compare To Zero  relop=>  OutDataTypeStr=uint8  ZeroCross=off
  Enabled Subsystem : Subsystem  TreatAsAtomicUnit=on
  Enabled Subsystem1 : Subsystem  TreatAsAtomicUnit=on
  Logical Operator : Logic  Operator=NOT  AllPortsSameDT=off  OutDataTypeStr=boolean
  Merge : Merge
  burst : Outport
  wires:
  Logical Operator/1 -> Enabled Subsystem/Enable
  Compare To Zero/1 -> Enabled Subsystem1/Enable, Logical Operator/1
  sel/1 -> Compare To Zero/1
  -p/1 -> Enabled Subsystem/1(In1)
  Enabled Subsystem/1(Out1) -> Merge/2
  Enabled Subsystem1/1(Out1) -> Merge/1
  p/1 -> Enabled Subsystem1/1(In1)
  Merge/1 -> burst/1

== system uwb_re_blackbox/Subsystem2/Transmit2/Spreading/Hop1/Kron1 ==
  p : Inport
  -p : Inport  Port=2
  sel : Inport  Port=3
  Compare To Zero : simulink/Logic and Bit Operations/Compare To Zero  relop=>  OutDataTypeStr=uint8  ZeroCross=off
  Enabled Subsystem : Subsystem  TreatAsAtomicUnit=on
  Enabled Subsystem1 : Subsystem  TreatAsAtomicUnit=on
  Logical Operator : Logic  Operator=NOT  AllPortsSameDT=off  OutDataTypeStr=boolean
  Merge : Merge
  burst : Outport
  wires:
  Merge/1 -> burst/1
  p/1 -> Enabled Subsystem1/1(In1)
  Enabled Subsystem1/1(Out1) -> Merge/1
  Enabled Subsystem/1(Out1) -> Merge/2
  -p/1 -> Enabled Subsystem/1(In1)
  sel/1 -> Compare To Zero/1
  Compare To Zero/1 -> Logical Operator/1, Enabled Subsystem1/Enable
  Logical Operator/1 -> Enabled Subsystem/Enable

== system uwb_re_blackbox/Subsystem2/Transmit2/Spreading/Hop1/Subsystem2 ==
  note: 16bit cua S mã hóa 1 cum xung gause 320 diem, them 7x320 diem 0
      | de tao ra 1/2 frame chua tin hieu
  In1 : Inport
  Buffer 48bit1 : Buffer  N=16
  Frame Conversion1 : FrameConversion
  Reshape3 : Reshape  OutputDimensionality=Customize  OutputDimensions=[320,1]
  Transpose1 : dspmtrx3/Transpose  Hermitian=off  overflowFlag=off
  Out1 : Outport
  wires:
  Frame Conversion1/1 -> Out1/1
  In1/1 -> Buffer 48bit1/1
  Reshape3/1 -> Frame Conversion1/1
  Transpose1/1 -> Reshape3/1
  Buffer 48bit1/1 -> Transpose1/1

== system uwb_re_blackbox/Subsystem2/Transmit2/Spreading/Hop1/Subsystem3 ==
  In1 : Inport
  Add1 : Sum  Inputs=+-
  Bi2De2 : commutil2/Bit to Integer Converter  nbits=2  bitOrder=MSB first  signedOutputValues=Unsigned  outDtype=int8  outDtypeSigned=Inherit via internal rule
  Gain2 : Gain  Gain=0.5  OutDataTypeStr=int8  RndMeth=Zero
  Gain4 : Gain  Gain=2  OutDataTypeStr=int8
  position : Outport
  sign : Outport  Port=2
  wires:
  Add1/1 -> position/1
  Bi2De2/1 -> Gain2/1, Add1/1
  Gain4/1 -> Add1/2
  Gain2/1 -> sign/1, Gain4/1
  In1/1 -> Bi2De2/1

== system uwb_re_blackbox/Subsystem2/Transmit2/Spreading/Hop1/Subsystem5 ==
  In1 : Inport
  matrix : Inport  Port=2
  CONST3 : Constant  Value=zeros(1,320)  VectorParams1D=off  OutDataTypeStr=int8  SampleTime=1
      settings: SamplingMode=Frame based
  Compare To Zero : simulink/Logic and Bit Operations/Compare To Zero  relop=>  OutDataTypeStr=uint8  ZeroCross=off
  Enabled Subsystem : Subsystem  TreatAsAtomicUnit=on
  Enabled Subsystem1 : Subsystem  TreatAsAtomicUnit=on
  Logical Operator : Logic  Operator=NOT  AllPortsSameDT=off  OutDataTypeStr=boolean
  Merge : Merge
  Reshape2 : Reshape  OutputDimensionality=Column vector (2-D)  OutputDimensions=[10,1]
  Out1 : Outport
  wires:
  Merge/1 -> Out1/1
  In1/1 -> Compare To Zero/1
  matrix/1 -> Enabled Subsystem/1(In1)
  Reshape2/1 -> Enabled Subsystem1/1(In1)
  Compare To Zero/1 -> Logical Operator/1, Enabled Subsystem1/Enable
  Enabled Subsystem1/1(Out1) -> Merge/1
  Enabled Subsystem/1(Out1) -> Merge/2
  Logical Operator/1 -> Enabled Subsystem/Enable
  CONST3/1 -> Reshape2/1

== system uwb_re_blackbox/Subsystem2/Transmit2/Spreading/Hop10/Kron ==
  p : Inport
  -p : Inport  Port=2
  sel : Inport  Port=3
  Compare To Zero : simulink/Logic and Bit Operations/Compare To Zero  relop=>  OutDataTypeStr=uint8  ZeroCross=off
  Enabled Subsystem : Subsystem  TreatAsAtomicUnit=on
  Enabled Subsystem1 : Subsystem  TreatAsAtomicUnit=on
  Logical Operator : Logic  Operator=NOT  AllPortsSameDT=off  OutDataTypeStr=boolean
  Merge : Merge
  burst : Outport
  wires:
  Merge/1 -> burst/1
  p/1 -> Enabled Subsystem1/1(In1)
  Enabled Subsystem1/1(Out1) -> Merge/1
  Enabled Subsystem/1(Out1) -> Merge/2
  -p/1 -> Enabled Subsystem/1(In1)
  sel/1 -> Compare To Zero/1
  Compare To Zero/1 -> Logical Operator/1, Enabled Subsystem1/Enable
  Logical Operator/1 -> Enabled Subsystem/Enable

== system uwb_re_blackbox/Subsystem2/Transmit2/Spreading/Hop10/Kron1 ==
  p : Inport
  -p : Inport  Port=2
  sel : Inport  Port=3
  Compare To Zero : simulink/Logic and Bit Operations/Compare To Zero  relop=>  OutDataTypeStr=uint8  ZeroCross=off
  Enabled Subsystem : Subsystem  TreatAsAtomicUnit=on
  Enabled Subsystem1 : Subsystem  TreatAsAtomicUnit=on
  Logical Operator : Logic  Operator=NOT  AllPortsSameDT=off  OutDataTypeStr=boolean
  Merge : Merge
  burst : Outport
  wires:
  Logical Operator/1 -> Enabled Subsystem/Enable
  Compare To Zero/1 -> Enabled Subsystem1/Enable, Logical Operator/1
  sel/1 -> Compare To Zero/1
  -p/1 -> Enabled Subsystem/1(In1)
  Enabled Subsystem/1(Out1) -> Merge/2
  Enabled Subsystem1/1(Out1) -> Merge/1
  p/1 -> Enabled Subsystem1/1(In1)
  Merge/1 -> burst/1

== system uwb_re_blackbox/Subsystem2/Transmit2/Spreading/Hop10/Subsystem2 ==
  note: 16bit cua S mã hóa 1 cum xung gause 320 diem, them 7x320 diem 0
      | de tao ra 1/2 frame chua tin hieu
  In1 : Inport
  Buffer 48bit1 : Buffer  N=16
  Frame Conversion1 : FrameConversion
  Reshape3 : Reshape  OutputDimensionality=Customize  OutputDimensions=[320,1]
  Transpose1 : dspmtrx3/Transpose  Hermitian=off  overflowFlag=off
  Out1 : Outport
  wires:
  Buffer 48bit1/1 -> Transpose1/1
  Transpose1/1 -> Reshape3/1
  Reshape3/1 -> Frame Conversion1/1
  In1/1 -> Buffer 48bit1/1
  Frame Conversion1/1 -> Out1/1

== system uwb_re_blackbox/Subsystem2/Transmit2/Spreading/Hop10/Subsystem3 ==
  In1 : Inport
  Add1 : Sum  Inputs=+-
  Bi2De2 : commutil2/Bit to Integer Converter  nbits=2  bitOrder=MSB first  signedOutputValues=Unsigned  outDtype=int8  outDtypeSigned=Inherit via internal rule
  Gain2 : Gain  Gain=0.5  OutDataTypeStr=int8  RndMeth=Zero
  Gain4 : Gain  Gain=2  OutDataTypeStr=int8
  position : Outport
  sign : Outport  Port=2
  wires:
  In1/1 -> Bi2De2/1
  Gain2/1 -> Gain4/1, sign/1
  Gain4/1 -> Add1/2
  Bi2De2/1 -> Add1/1, Gain2/1
  Add1/1 -> position/1

== system uwb_re_blackbox/Subsystem2/Transmit2/Spreading/Hop10/Subsystem5 ==
  In1 : Inport
  matrix : Inport  Port=2
  CONST3 : Constant  Value=zeros(1,320)  VectorParams1D=off  OutDataTypeStr=int8  SampleTime=1
      settings: SamplingMode=Frame based
  Compare To Zero : simulink/Logic and Bit Operations/Compare To Zero  relop=>  OutDataTypeStr=uint8  ZeroCross=off
  Enabled Subsystem : Subsystem  TreatAsAtomicUnit=on
  Enabled Subsystem1 : Subsystem  TreatAsAtomicUnit=on
  Logical Operator : Logic  Operator=NOT  AllPortsSameDT=off  OutDataTypeStr=boolean
  Merge : Merge
  Reshape2 : Reshape  OutputDimensionality=Column vector (2-D)  OutputDimensions=[10,1]
  Out1 : Outport
  wires:
  CONST3/1 -> Reshape2/1
  Logical Operator/1 -> Enabled Subsystem/Enable
  Enabled Subsystem/1(Out1) -> Merge/2
  Enabled Subsystem1/1(Out1) -> Merge/1
  Compare To Zero/1 -> Enabled Subsystem1/Enable, Logical Operator/1
  Reshape2/1 -> Enabled Subsystem1/1(In1)
  matrix/1 -> Enabled Subsystem/1(In1)
  In1/1 -> Compare To Zero/1
  Merge/1 -> Out1/1
